simulink model "model_InputConditioningAutoRestart_Test"  (R2024a)
settings: Solver=VariableStepAuto  StartTime=0.0  StopTime=10.0  RelTol=1e-3
settings Model: Creator=Gabriel  LastModifiedBy=Gabriel

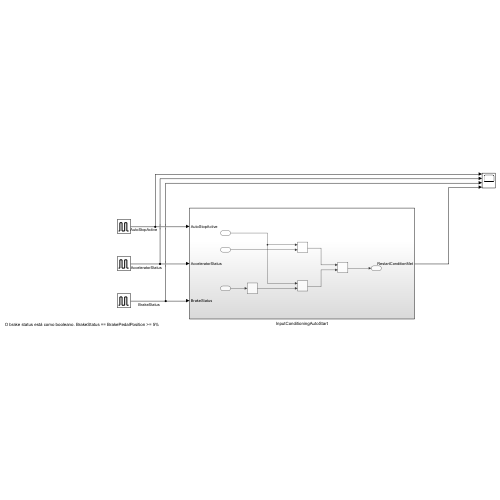
[thumbnail: Simulink's stored preview of the top-level diagram]
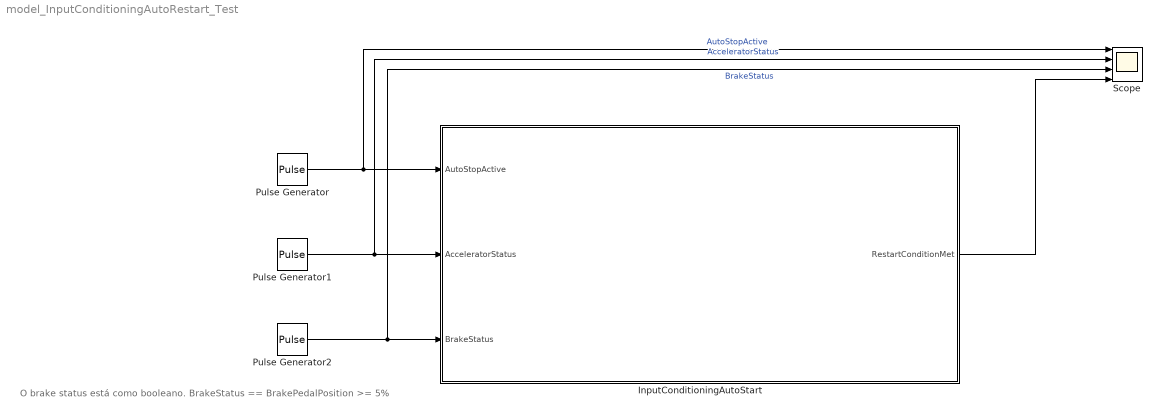
== system model_InputConditioningAutoRestart_Test ==
  note: O brake status está como booleano. BrakeStatus == BrakePedalPosition >= 5%
  InputConditioningAutoStart : Subsystem
  Pulse Generator : DiscretePulseGenerator  PulseType=Time based  PulseWidth=60
  Pulse Generator1 : DiscretePulseGenerator  PulseType=Time based  PulseWidth=20
  Pulse Generator2 : DiscretePulseGenerator  PulseType=Time based  PulseWidth=45
  Scope : Scope  NumInputPorts=4
  wires:
  Pulse Generator/1 -> Scope/1, InputConditioningAutoStart/1(AutoStopActive)  "AutoStopActive"
  Pulse Generator1/1 -> Scope/2, InputConditioningAutoStart/2(AcceleratorStatus)  "AcceleratorStatus"
  Pulse Generator2/1 -> Scope/3, InputConditioningAutoStart/3(BrakeStatus)  "BrakeStatus"
  InputConditioningAutoStart/1(RestartConditionMet) -> Scope/4

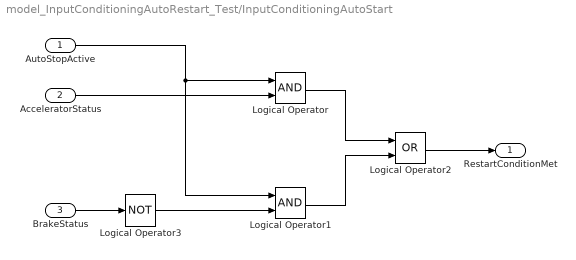
== system model_InputConditioningAutoRestart_Test/InputConditioningAutoStart ==
  AutoStopActive : Inport
  AcceleratorStatus : Inport  Port=2
  BrakeStatus : Inport  Port=3
  Logical Operator : Logic  AllPortsSameDT=off  OutDataTypeStr=boolean
  Logical Operator1 : Logic  AllPortsSameDT=off  OutDataTypeStr=boolean
  Logical Operator2 : Logic  Operator=OR  AllPortsSameDT=off  OutDataTypeStr=boolean
  Logical Operator3 : Logic  Operator=NOT  AllPortsSameDT=off  OutDataTypeStr=boolean
  RestartConditionMet : Outport
  wires:
  AcceleratorStatus/1 -> Logical Operator/2
  AutoStopActive/1 -> Logical Operator1/1, Logical Operator/1
  BrakeStatus/1 -> Logical Operator3/1
  Logical Operator/1 -> Logical Operator2/1
  Logical Operator1/1 -> Logical Operator2/2
  Logical Operator2/1 -> RestartConditionMet/1
  Logical Operator3/1 -> Logical Operator1/2
